simulink model "SecRwLtStLgrstUpwdDnwdIsPosChk"  (R2024b)
settings: Solver=FixedStepDiscrete  StartTime=0.0  StopTime=10.0  FixedStep=0.01  RelTol=1e-3
undefined symbols (not defined in the file or in its folder): KeSMSuSecRwStLegrestUpwdDwnwdPosDelta_Val, KeSMSuSecRwStLegrestUpwdDwnwdPosTolr_Val
libraries: StIsPosChkLib x13, simulink x7
(part 2 of 2)

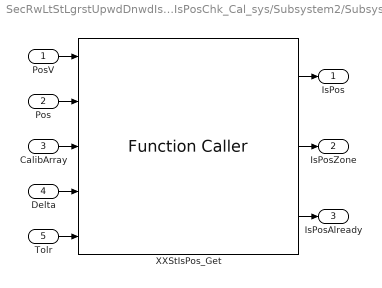
== system SecRwLtStLgrstUpwdDnwdIsPosChk/SecRwLtStLgrstUpwdDnwdIsPosChk_Cal_sys/Subsystem2/Subsystem11 ==
  PosV : Inport
  Pos : Inport  Port=2
  CalibArray : Inport  Port=3
  Delta : Inport  Port=4
  Tolr : Inport  Port=5
  XXStIsPos_Get : FunctionCaller  FunctionPrototype=[IsPos,IsPosZone,IsPosAlready] = XXStIsPos_Get(PosV,Pos,CalibArray,Delta,Tolr)  InputArgumentSpecifications=boolean(true), uint16(1), uint16([1;1;1]), uint16(1), uint16(1)  OutputArgumentSpecifications=boolean(true), boolean(true), boolean(true)
  IsPos : Outport  VectorParamsAs1DForOutWhenUnconnected=off
  IsPosZone : Outport  Port=2  VectorParamsAs1DForOutWhenUnconnected=off
  IsPosAlready : Outport  Port=3  VectorParamsAs1DForOutWhenUnconnected=off
  wires:
  PosV/1 -> XXStIsPos_Get/1
  Delta/1 -> XXStIsPos_Get/4
  Pos/1 -> XXStIsPos_Get/2
  CalibArray/1 -> XXStIsPos_Get/3
  XXStIsPos_Get/2 -> IsPosZone/1
  Tolr/1 -> XXStIsPos_Get/5
  XXStIsPos_Get/3 -> IsPosAlready/1
  XXStIsPos_Get/1 -> IsPos/1

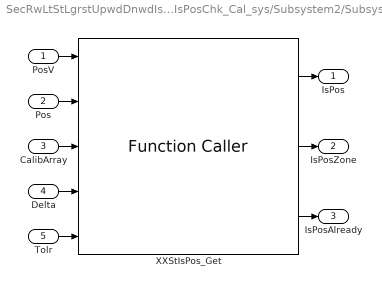
== system SecRwLtStLgrstUpwdDnwdIsPosChk/SecRwLtStLgrstUpwdDnwdIsPosChk_Cal_sys/Subsystem2/Subsystem12 ==
  PosV : Inport
  Pos : Inport  Port=2
  CalibArray : Inport  Port=3
  Delta : Inport  Port=4
  Tolr : Inport  Port=5
  XXStIsPos_Get : FunctionCaller  FunctionPrototype=[IsPos,IsPosZone,IsPosAlready] = XXStIsPos_Get(PosV,Pos,CalibArray,Delta,Tolr)  InputArgumentSpecifications=boolean(true), uint16(1), uint16([1;1;1]), uint16(1), uint16(1)  OutputArgumentSpecifications=boolean(true), boolean(true), boolean(true)
  IsPos : Outport  VectorParamsAs1DForOutWhenUnconnected=off
  IsPosZone : Outport  Port=2  VectorParamsAs1DForOutWhenUnconnected=off
  IsPosAlready : Outport  Port=3  VectorParamsAs1DForOutWhenUnconnected=off
  wires:
  XXStIsPos_Get/1 -> IsPos/1
  XXStIsPos_Get/3 -> IsPosAlready/1
  Tolr/1 -> XXStIsPos_Get/5
  XXStIsPos_Get/2 -> IsPosZone/1
  CalibArray/1 -> XXStIsPos_Get/3
  Pos/1 -> XXStIsPos_Get/2
  Delta/1 -> XXStIsPos_Get/4
  PosV/1 -> XXStIsPos_Get/1

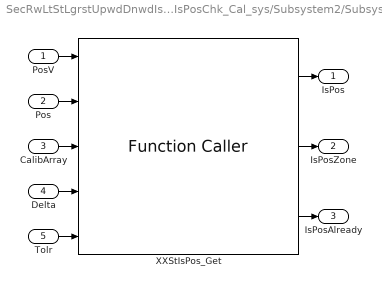
== system SecRwLtStLgrstUpwdDnwdIsPosChk/SecRwLtStLgrstUpwdDnwdIsPosChk_Cal_sys/Subsystem2/Subsystem13 ==
  PosV : Inport
  Pos : Inport  Port=2
  CalibArray : Inport  Port=3
  Delta : Inport  Port=4
  Tolr : Inport  Port=5
  XXStIsPos_Get : FunctionCaller  FunctionPrototype=[IsPos,IsPosZone,IsPosAlready] = XXStIsPos_Get(PosV,Pos,CalibArray,Delta,Tolr)  InputArgumentSpecifications=boolean(true), uint16(1), uint16([1;1;1]), uint16(1), uint16(1)  OutputArgumentSpecifications=boolean(true), boolean(true), boolean(true)
  IsPos : Outport  VectorParamsAs1DForOutWhenUnconnected=off
  IsPosZone : Outport  Port=2  VectorParamsAs1DForOutWhenUnconnected=off
  IsPosAlready : Outport  Port=3  VectorParamsAs1DForOutWhenUnconnected=off
  wires:
  PosV/1 -> XXStIsPos_Get/1
  Delta/1 -> XXStIsPos_Get/4
  Pos/1 -> XXStIsPos_Get/2
  CalibArray/1 -> XXStIsPos_Get/3
  XXStIsPos_Get/2 -> IsPosZone/1
  Tolr/1 -> XXStIsPos_Get/5
  XXStIsPos_Get/3 -> IsPosAlready/1
  XXStIsPos_Get/1 -> IsPos/1

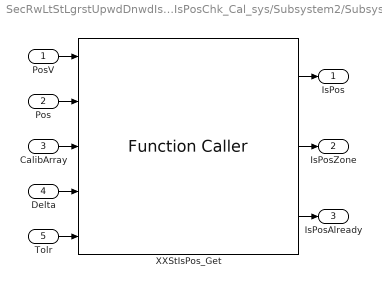
== system SecRwLtStLgrstUpwdDnwdIsPosChk/SecRwLtStLgrstUpwdDnwdIsPosChk_Cal_sys/Subsystem2/Subsystem14 ==
  PosV : Inport
  Pos : Inport  Port=2
  CalibArray : Inport  Port=3
  Delta : Inport  Port=4
  Tolr : Inport  Port=5
  XXStIsPos_Get : FunctionCaller  FunctionPrototype=[IsPos,IsPosZone,IsPosAlready] = XXStIsPos_Get(PosV,Pos,CalibArray,Delta,Tolr)  InputArgumentSpecifications=boolean(true), uint16(1), uint16([1;1;1]), uint16(1), uint16(1)  OutputArgumentSpecifications=boolean(true), boolean(true), boolean(true)
  IsPos : Outport  VectorParamsAs1DForOutWhenUnconnected=off
  IsPosZone : Outport  Port=2  VectorParamsAs1DForOutWhenUnconnected=off
  IsPosAlready : Outport  Port=3  VectorParamsAs1DForOutWhenUnconnected=off
  wires:
  XXStIsPos_Get/1 -> IsPos/1
  XXStIsPos_Get/3 -> IsPosAlready/1
  Tolr/1 -> XXStIsPos_Get/5
  XXStIsPos_Get/2 -> IsPosZone/1
  CalibArray/1 -> XXStIsPos_Get/3
  Pos/1 -> XXStIsPos_Get/2
  Delta/1 -> XXStIsPos_Get/4
  PosV/1 -> XXStIsPos_Get/1

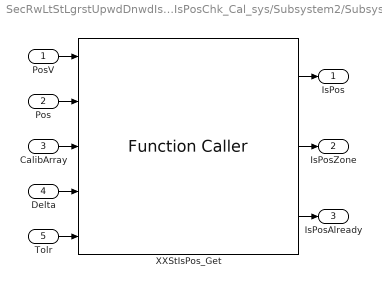
== system SecRwLtStLgrstUpwdDnwdIsPosChk/SecRwLtStLgrstUpwdDnwdIsPosChk_Cal_sys/Subsystem2/Subsystem15 ==
  PosV : Inport
  Pos : Inport  Port=2
  CalibArray : Inport  Port=3
  Delta : Inport  Port=4
  Tolr : Inport  Port=5
  XXStIsPos_Get : FunctionCaller  FunctionPrototype=[IsPos,IsPosZone,IsPosAlready] = XXStIsPos_Get(PosV,Pos,CalibArray,Delta,Tolr)  InputArgumentSpecifications=boolean(true), uint16(1), uint16([1;1;1]), uint16(1), uint16(1)  OutputArgumentSpecifications=boolean(true), boolean(true), boolean(true)
  IsPos : Outport  VectorParamsAs1DForOutWhenUnconnected=off
  IsPosZone : Outport  Port=2  VectorParamsAs1DForOutWhenUnconnected=off
  IsPosAlready : Outport  Port=3  VectorParamsAs1DForOutWhenUnconnected=off
  wires:
  PosV/1 -> XXStIsPos_Get/1
  Delta/1 -> XXStIsPos_Get/4
  Pos/1 -> XXStIsPos_Get/2
  CalibArray/1 -> XXStIsPos_Get/3
  XXStIsPos_Get/2 -> IsPosZone/1
  Tolr/1 -> XXStIsPos_Get/5
  XXStIsPos_Get/3 -> IsPosAlready/1
  XXStIsPos_Get/1 -> IsPos/1

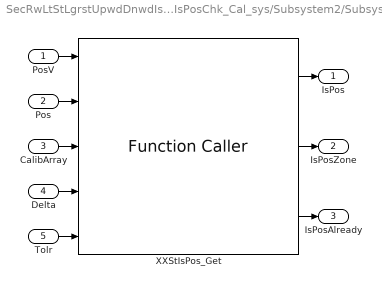
== system SecRwLtStLgrstUpwdDnwdIsPosChk/SecRwLtStLgrstUpwdDnwdIsPosChk_Cal_sys/Subsystem2/Subsystem2 ==
  PosV : Inport
  Pos : Inport  Port=2
  CalibArray : Inport  Port=3
  Delta : Inport  Port=4
  Tolr : Inport  Port=5
  XXStIsPos_Get : FunctionCaller  FunctionPrototype=[IsPos,IsPosZone,IsPosAlready] = XXStIsPos_Get(PosV,Pos,CalibArray,Delta,Tolr)  InputArgumentSpecifications=boolean(true), uint16(1), uint16([1;1;1]), uint16(1), uint16(1)  OutputArgumentSpecifications=boolean(true), boolean(true), boolean(true)
  IsPos : Outport  VectorParamsAs1DForOutWhenUnconnected=off
  IsPosZone : Outport  Port=2  VectorParamsAs1DForOutWhenUnconnected=off
  IsPosAlready : Outport  Port=3  VectorParamsAs1DForOutWhenUnconnected=off
  wires:
  PosV/1 -> XXStIsPos_Get/1
  Delta/1 -> XXStIsPos_Get/4
  Pos/1 -> XXStIsPos_Get/2
  CalibArray/1 -> XXStIsPos_Get/3
  XXStIsPos_Get/2 -> IsPosZone/1
  Tolr/1 -> XXStIsPos_Get/5
  XXStIsPos_Get/3 -> IsPosAlready/1
  XXStIsPos_Get/1 -> IsPos/1

== system SecRwLtStLgrstUpwdDnwdIsPosChk/SecRwLtStLgrstUpwdDnwdIsPosChk_Cal_sys/Subsystem2/Subsystem3 ==
  PosV : Inport
  Pos : Inport  Port=2
  CalibArray : Inport  Port=3
  Delta : Inport  Port=4
  Tolr : Inport  Port=5
  XXStIsPos_Get : FunctionCaller  FunctionPrototype=[IsPos,IsPosZone,IsPosAlready] = XXStIsPos_Get(PosV,Pos,CalibArray,Delta,Tolr)  InputArgumentSpecifications=boolean(true), uint16(1), uint16([1;1;1]), uint16(1), uint16(1)  OutputArgumentSpecifications=boolean(true), boolean(true), boolean(true)
  IsPos : Outport  VectorParamsAs1DForOutWhenUnconnected=off
  IsPosZone : Outport  Port=2  VectorParamsAs1DForOutWhenUnconnected=off
  IsPosAlready : Outport  Port=3  VectorParamsAs1DForOutWhenUnconnected=off
  wires:
  PosV/1 -> XXStIsPos_Get/1
  Delta/1 -> XXStIsPos_Get/4
  Pos/1 -> XXStIsPos_Get/2
  CalibArray/1 -> XXStIsPos_Get/3
  XXStIsPos_Get/2 -> IsPosZone/1
  Tolr/1 -> XXStIsPos_Get/5
  XXStIsPos_Get/3 -> IsPosAlready/1
  XXStIsPos_Get/1 -> IsPos/1

== system SecRwLtStLgrstUpwdDnwdIsPosChk/SecRwLtStLgrstUpwdDnwdIsPosChk_Cal_sys/Subsystem2/Subsystem4 ==
  PosV : Inport
  Pos : Inport  Port=2
  CalibArray : Inport  Port=3
  Delta : Inport  Port=4
  Tolr : Inport  Port=5
  XXStIsPos_Get : FunctionCaller  FunctionPrototype=[IsPos,IsPosZone,IsPosAlready] = XXStIsPos_Get(PosV,Pos,CalibArray,Delta,Tolr)  InputArgumentSpecifications=boolean(true), uint16(1), uint16([1;1;1]), uint16(1), uint16(1)  OutputArgumentSpecifications=boolean(true), boolean(true), boolean(true)
  IsPos : Outport  VectorParamsAs1DForOutWhenUnconnected=off
  IsPosZone : Outport  Port=2  VectorParamsAs1DForOutWhenUnconnected=off
  IsPosAlready : Outport  Port=3  VectorParamsAs1DForOutWhenUnconnected=off
  wires:
  PosV/1 -> XXStIsPos_Get/1
  Delta/1 -> XXStIsPos_Get/4
  Pos/1 -> XXStIsPos_Get/2
  CalibArray/1 -> XXStIsPos_Get/3
  XXStIsPos_Get/2 -> IsPosZone/1
  Tolr/1 -> XXStIsPos_Get/5
  XXStIsPos_Get/3 -> IsPosAlready/1
  XXStIsPos_Get/1 -> IsPos/1

== system SecRwLtStLgrstUpwdDnwdIsPosChk/SecRwLtStLgrstUpwdDnwdIsPosChk_Cal_sys/Subsystem2/Subsystem5 ==
  PosV : Inport
  Pos : Inport  Port=2
  CalibArray : Inport  Port=3
  Delta : Inport  Port=4
  Tolr : Inport  Port=5
  XXStIsPos_Get : FunctionCaller  FunctionPrototype=[IsPos,IsPosZone,IsPosAlready] = XXStIsPos_Get(PosV,Pos,CalibArray,Delta,Tolr)  InputArgumentSpecifications=boolean(true), uint16(1), uint16([1;1;1]), uint16(1), uint16(1)  OutputArgumentSpecifications=boolean(true), boolean(true), boolean(true)
  IsPos : Outport  VectorParamsAs1DForOutWhenUnconnected=off
  IsPosZone : Outport  Port=2  VectorParamsAs1DForOutWhenUnconnected=off
  IsPosAlready : Outport  Port=3  VectorParamsAs1DForOutWhenUnconnected=off
  wires:
  PosV/1 -> XXStIsPos_Get/1
  Delta/1 -> XXStIsPos_Get/4
  Pos/1 -> XXStIsPos_Get/2
  CalibArray/1 -> XXStIsPos_Get/3
  XXStIsPos_Get/2 -> IsPosZone/1
  Tolr/1 -> XXStIsPos_Get/5
  XXStIsPos_Get/3 -> IsPosAlready/1
  XXStIsPos_Get/1 -> IsPos/1

== system SecRwLtStLgrstUpwdDnwdIsPosChk/SecRwLtStLgrstUpwdDnwdIsPosChk_Cal_sys/Subsystem2/Subsystem6 ==
  PosV : Inport
  Pos : Inport  Port=2
  CalibArray : Inport  Port=3
  Delta : Inport  Port=4
  Tolr : Inport  Port=5
  XXStIsPos_Get : FunctionCaller  FunctionPrototype=[IsPos,IsPosZone,IsPosAlready] = XXStIsPos_Get(PosV,Pos,CalibArray,Delta,Tolr)  InputArgumentSpecifications=boolean(true), uint16(1), uint16([1;1;1]), uint16(1), uint16(1)  OutputArgumentSpecifications=boolean(true), boolean(true), boolean(true)
  IsPos : Outport  VectorParamsAs1DForOutWhenUnconnected=off
  IsPosZone : Outport  Port=2  VectorParamsAs1DForOutWhenUnconnected=off
  IsPosAlready : Outport  Port=3  VectorParamsAs1DForOutWhenUnconnected=off
  wires:
  PosV/1 -> XXStIsPos_Get/1
  Delta/1 -> XXStIsPos_Get/4
  Pos/1 -> XXStIsPos_Get/2
  CalibArray/1 -> XXStIsPos_Get/3
  XXStIsPos_Get/2 -> IsPosZone/1
  Tolr/1 -> XXStIsPos_Get/5
  XXStIsPos_Get/3 -> IsPosAlready/1
  XXStIsPos_Get/1 -> IsPos/1

== system SecRwLtStLgrstUpwdDnwdIsPosChk/SecRwLtStLgrstUpwdDnwdIsPosChk_Cal_sys/Subsystem2/Subsystem7 ==
  PosV : Inport
  Pos : Inport  Port=2
  CalibArray : Inport  Port=3
  Delta : Inport  Port=4
  Tolr : Inport  Port=5
  XXStIsPos_Get : FunctionCaller  FunctionPrototype=[IsPos,IsPosZone,IsPosAlready] = XXStIsPos_Get(PosV,Pos,CalibArray,Delta,Tolr)  InputArgumentSpecifications=boolean(true), uint16(1), uint16([1;1;1]), uint16(1), uint16(1)  OutputArgumentSpecifications=boolean(true), boolean(true), boolean(true)
  IsPos : Outport  VectorParamsAs1DForOutWhenUnconnected=off
  IsPosZone : Outport  Port=2  VectorParamsAs1DForOutWhenUnconnected=off
  IsPosAlready : Outport  Port=3  VectorParamsAs1DForOutWhenUnconnected=off
  wires:
  PosV/1 -> XXStIsPos_Get/1
  Delta/1 -> XXStIsPos_Get/4
  Pos/1 -> XXStIsPos_Get/2
  CalibArray/1 -> XXStIsPos_Get/3
  XXStIsPos_Get/2 -> IsPosZone/1
  Tolr/1 -> XXStIsPos_Get/5
  XXStIsPos_Get/3 -> IsPosAlready/1
  XXStIsPos_Get/1 -> IsPos/1

== system SecRwLtStLgrstUpwdDnwdIsPosChk/SecRwLtStLgrstUpwdDnwdIsPosChk_Cal_sys/Subsystem2/Subsystem8 ==
  PosV : Inport
  Pos : Inport  Port=2
  CalibArray : Inport  Port=3
  Delta : Inport  Port=4
  Tolr : Inport  Port=5
  XXStIsPos_Get : FunctionCaller  FunctionPrototype=[IsPos,IsPosZone,IsPosAlready] = XXStIsPos_Get(PosV,Pos,CalibArray,Delta,Tolr)  InputArgumentSpecifications=boolean(true), uint16(1), uint16([1;1;1]), uint16(1), uint16(1)  OutputArgumentSpecifications=boolean(true), boolean(true), boolean(true)
  IsPos : Outport  VectorParamsAs1DForOutWhenUnconnected=off
  IsPosZone : Outport  Port=2  VectorParamsAs1DForOutWhenUnconnected=off
  IsPosAlready : Outport  Port=3  VectorParamsAs1DForOutWhenUnconnected=off
  wires:
  PosV/1 -> XXStIsPos_Get/1
  Delta/1 -> XXStIsPos_Get/4
  Pos/1 -> XXStIsPos_Get/2
  CalibArray/1 -> XXStIsPos_Get/3
  XXStIsPos_Get/2 -> IsPosZone/1
  Tolr/1 -> XXStIsPos_Get/5
  XXStIsPos_Get/3 -> IsPosAlready/1
  XXStIsPos_Get/1 -> IsPos/1

== system SecRwLtStLgrstUpwdDnwdIsPosChk/SecRwLtStLgrstUpwdDnwdIsPosChk_Cal_sys/Subsystem2/Subsystem9 ==
  PosV : Inport
  Pos : Inport  Port=2
  CalibArray : Inport  Port=3
  Delta : Inport  Port=4
  Tolr : Inport  Port=5
  XXStIsPos_Get : FunctionCaller  FunctionPrototype=[IsPos,IsPosZone,IsPosAlready] = XXStIsPos_Get(PosV,Pos,CalibArray,Delta,Tolr)  InputArgumentSpecifications=boolean(true), uint16(1), uint16([1;1;1]), uint16(1), uint16(1)  OutputArgumentSpecifications=boolean(true), boolean(true), boolean(true)
  IsPos : Outport  VectorParamsAs1DForOutWhenUnconnected=off
  IsPosZone : Outport  Port=2  VectorParamsAs1DForOutWhenUnconnected=off
  IsPosAlready : Outport  Port=3  VectorParamsAs1DForOutWhenUnconnected=off
  wires:
  XXStIsPos_Get/1 -> IsPos/1
  XXStIsPos_Get/3 -> IsPosAlready/1
  Tolr/1 -> XXStIsPos_Get/5
  XXStIsPos_Get/2 -> IsPosZone/1
  CalibArray/1 -> XXStIsPos_Get/3
  Pos/1 -> XXStIsPos_Get/2
  Delta/1 -> XXStIsPos_Get/4
  PosV/1 -> XXStIsPos_Get/1
